simulink model "elec_angle_id"  (R2023a)
settings: configuration reference "config" (kept outside this file)
settings Model: DataDictionary=model_config.sldd  Creator=huangcheng  LastModifiedBy=Administrator
settings ConfigSetRef: SourceName=config

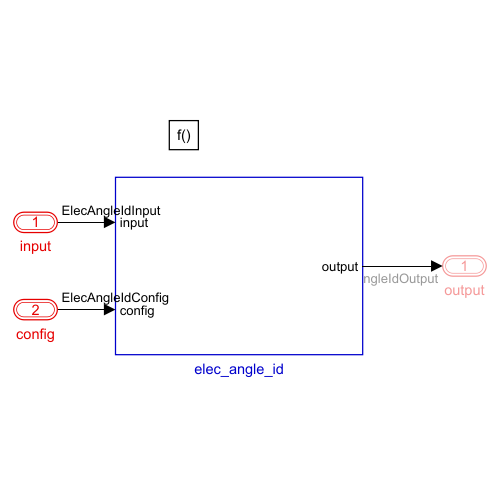
[thumbnail: Simulink's stored preview of the top-level diagram]
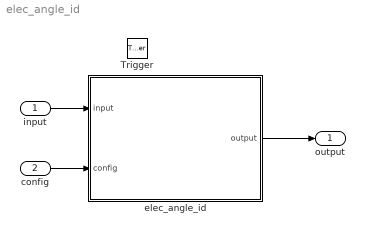
== system elec_angle_id ==
  input : Inport  OutDataTypeStr=Bus: ElecAngleIdInput  BusOutputAsStruct=on
  config : Inport  Port=2  OutDataTypeStr=Bus: ElecAngleIdConfig  BusOutputAsStruct=on
  Trigger : TriggerPort  TriggerType=function-call  VariantControl=(inherit)  PortDimensions=1
  elec_angle_id : Subsystem  SystemSampleTime=10e-5
  output : Outport  OutDataTypeStr=Bus: ElecAngleIdOutput  BusOutputAsStruct=on
      settings: EnsureOutportIsVirtual=on
  wires:
  config/1 -> elec_angle_id/2(config)
  input/1 -> elec_angle_id/1(input)
  elec_angle_id/1(output) -> output/1

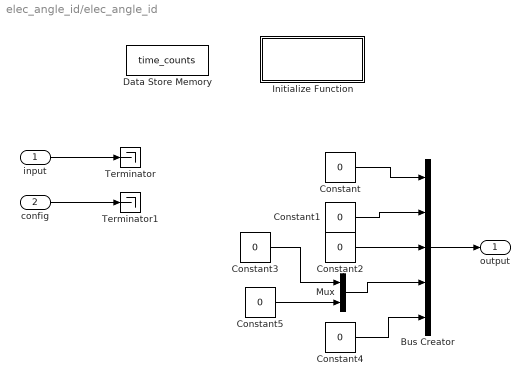
== system elec_angle_id/elec_angle_id ==
  input : Inport
  config : Inport  Port=2
  Bus Creator : BusCreator  Inputs=5  OutDataTypeStr=Bus: ElecAngleIdOutput  NonVirtualBus=on
      settings: InheritFromInputs=off
  Constant{,1,3,5} (4 alike) : Constant  Value=0  OutDataTypeStr=single
  Constant2 : Constant  Value=0  OutDataTypeStr=int8
  Constant4 : Constant  Value=0  OutDataTypeStr=uint8
  Data Store Memory : DataStoreMemory  DataStoreName=time_counts  WriteAfterWriteMsg=warning  ShowAdditionalParam=off  OutDataTypeStr=single
  Initialize Function : Subsystem  TreatAsAtomicUnit=on
  Mux : Mux  Inputs=2
  Terminator : Terminator
  Terminator1 : Terminator
  output : Outport
  wires:
  input/1 -> Terminator/1
  Constant4/1 -> Bus Creator/5
  Constant/1 -> Bus Creator/1
  config/1 -> Terminator1/1
  Constant1/1 -> Bus Creator/2
  Constant2/1 -> Bus Creator/3
  Bus Creator/1 -> output/1
  Mux/1 -> Bus Creator/4
  Constant3/1 -> Mux/1
  Constant5/1 -> Mux/2

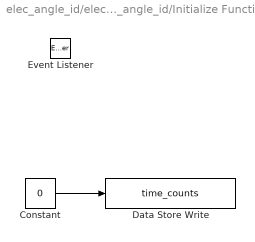
== system elec_angle_id/elec_angle_id/Initialize Function ==
  Constant : Constant  Value=0  OutDataTypeStr=single
  Data Store Write : DataStoreWrite  DataStoreName=time_counts  IndexOptions=Index vector (dialog)  Indices=1  OutputSizes=1
  Event Listener : EventListener  DisableCoverage=on  EventName=reset
  wires:
  Constant/1 -> Data Store Write/1
